simulink model "P1s1"  (R2015b)
settings: Solver=VariableStepAuto  StartTime=0.0  StopTime=10.0  RelTol=1e-3
settings Model: Creator=xmax1946  LastModifiedBy=xmax1946

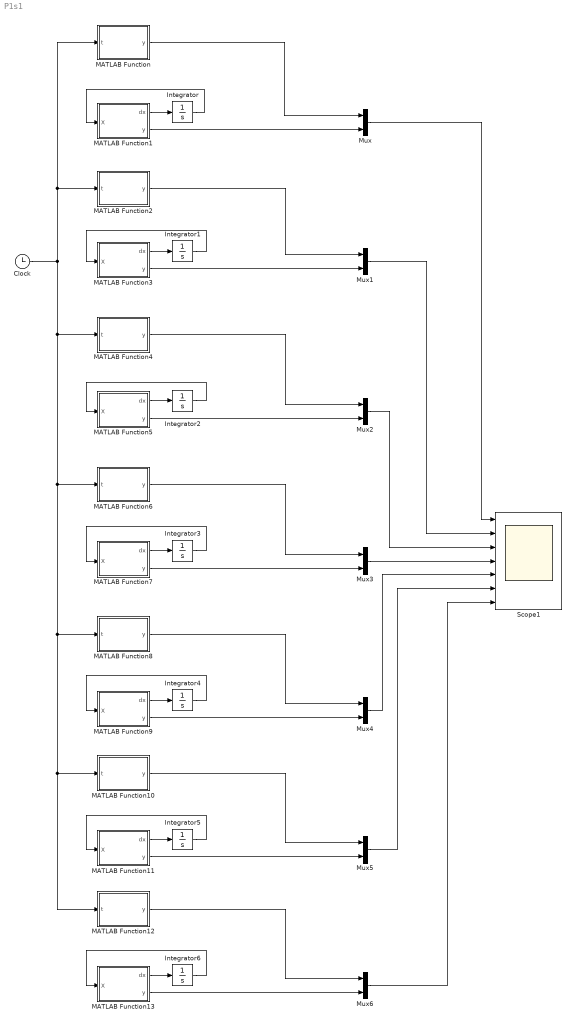
== system P1s1 ==
  Clock : Clock
  Integrator{,1..4} (5 alike) : Integrator  InitialCondition=[1;1]
  Integrator5 : Integrator  InitialCondition=[1;1;1]
  Integrator6 : Integrator  InitialCondition=[1;1;1]
  MATLAB Function : MATLAB Function  TreatAsAtomicUnit=on
  MATLAB Function1 : MATLAB Function  TreatAsAtomicUnit=on
  MATLAB Function10 : MATLAB Function  TreatAsAtomicUnit=on
  MATLAB Function11 : MATLAB Function  TreatAsAtomicUnit=on
  MATLAB Function12 : MATLAB Function  TreatAsAtomicUnit=on
  MATLAB Function13 : MATLAB Function  TreatAsAtomicUnit=on
  MATLAB Function2 : MATLAB Function  TreatAsAtomicUnit=on
  MATLAB Function3 : MATLAB Function  TreatAsAtomicUnit=on
  MATLAB Function4 : MATLAB Function  TreatAsAtomicUnit=on
  MATLAB Function5 : MATLAB Function  TreatAsAtomicUnit=on
  MATLAB Function6 : MATLAB Function  TreatAsAtomicUnit=on
  MATLAB Function7 : MATLAB Function  TreatAsAtomicUnit=on
  MATLAB Function8 : MATLAB Function  TreatAsAtomicUnit=on
  MATLAB Function9 : MATLAB Function  TreatAsAtomicUnit=on
  Mux{,1..6} (7 alike) : Mux  Inputs=2
  Scope1 : Scope  NumInputPorts=7
  wires:
  Integrator/1 -> MATLAB Function1/1(X)
  Clock/1 -> MATLAB Function12/1(t), MATLAB Function10/1(t), MATLAB Function8/1(t), MATLAB Function6/1(t), MATLAB Function4/1(t), MATLAB Function2/1(t), MATLAB Function/1(t)
  MATLAB Function1/1(dx) -> Integrator/1
  MATLAB Function3/1(dx) -> Integrator1/1
  Integrator1/1 -> MATLAB Function3/1(X)
  Mux/1 -> Scope1/1
  MATLAB Function3/2(y) -> Mux1/2
  MATLAB Function2/1(y) -> Mux1/1
  MATLAB Function1/2(y) -> Mux/2
  MATLAB Function/1(y) -> Mux/1
  Mux1/1 -> Scope1/2
  MATLAB Function5/1(dx) -> Integrator2/1
  Integrator2/1 -> MATLAB Function5/1(X)
  MATLAB Function5/2(y) -> Mux2/2
  MATLAB Function4/1(y) -> Mux2/1
  Mux2/1 -> Scope1/3
  MATLAB Function7/1(dx) -> Integrator3/1
  Integrator3/1 -> MATLAB Function7/1(X)
  MATLAB Function7/2(y) -> Mux3/2
  MATLAB Function6/1(y) -> Mux3/1
  Mux3/1 -> Scope1/4
  MATLAB Function9/1(dx) -> Integrator4/1
  Integrator4/1 -> MATLAB Function9/1(X)
  MATLAB Function9/2(y) -> Mux4/2
  MATLAB Function8/1(y) -> Mux4/1
  Mux4/1 -> Scope1/5
  MATLAB Function11/1(dx) -> Integrator5/1
  Integrator5/1 -> MATLAB Function11/1(X)
  MATLAB Function11/2(y) -> Mux5/2
  MATLAB Function10/1(y) -> Mux5/1
  Mux5/1 -> Scope1/6
  MATLAB Function13/1(dx) -> Integrator6/1
  Integrator6/1 -> MATLAB Function13/1(X)
  MATLAB Function13/2(y) -> Mux6/2
  MATLAB Function12/1(y) -> Mux6/1
  Mux6/1 -> Scope1/7

== matlab function P1s1/MATLAB Function1 ==
  data: dx output; X input; y output
function [dx,y] = fcn1(X)

A=[1,-1;0,-1];
B=[1;1];
C=[1,2];
u=1;
dx=A*X+B*u;
y=C*X;

== matlab function P1s1/MATLAB Function ==
  data: t input; y output
function y = f1(t)
y = exp(t)+2;

== matlab function P1s1/MATLAB Function2 ==
  data: t input; y output
function y = f2(t)
y = 11/4 - (25*exp(-4*t))/12 - (2*exp(-t))/3;

== matlab function P1s1/MATLAB Function3 ==
  data: dx output; X input; y output
function [dx,y] = fcn2(X)

A=[0,1;-4,-5];
B=[1;2];
C=[1,-1];
u=1;
dx=A*X+B*u;
y=C*X;

== matlab function P1s1/MATLAB Function4 ==
  data: t input; y output
function y = f3(t)
y = t*exp(-3*t) - (4*exp(-3*t))/3 + 10/3;

== matlab function P1s1/MATLAB Function5 ==
  data: dx output; X input; y output
function [dx,y] = fcn3(X)

A=[-3,1;0,-3];
B=[1;0];
C=[1,1];
u=10;
dx=A*X+B*u;
y=C*X;

== matlab function P1s1/MATLAB Function6 ==
  data: t input; y output
function y = f4(t)
y =5/3 - exp(-4*t) - (2*exp(-3*t))/3;

== matlab function P1s1/MATLAB Function7 ==
  data: dx output; X input; y output
function [dx,y] = fcn4(X)

A=[-4,0;0,-3];
B=[0;1];
C=[-1,1];
u=5;
dx=A*X+B*u;
y=C*X;

== matlab function P1s1/MATLAB Function8 ==
  data: t input; y output
function y = f5(t)
y =33*exp(-t) - 12*exp(-2*t) - 20;

== matlab function P1s1/MATLAB Function9 ==
  data: dx output; X input; y output
function [dx,y] = fcn5(X)

A=[0,1;-2,-3];
B=[1;1];
C=[1,0];
u=-10;
dx=A*X+B*u;
y=C*X;

== matlab function P1s1/MATLAB Function10 ==
  data: t input; y output
function y = f6(t)
y =1 - exp(-2*t);

== matlab function P1s1/MATLAB Function11 ==
  data: dx output; X input; y output
function [dx,y] = fcn6(X)

A=[-1,0,0;0,-2,1;0,0,-2];
B=[1;1;0];
C=[1,0,-1];
u=1;
dx=A*X+B*u;
y=C*X;

== matlab function P1s1/MATLAB Function12 ==
  data: t input; y output
function y = f7(t)
y =(219*exp(-5*t))/125 + (44*t*exp(-5*t))/25 + (2*t^2*exp(-5*t))/5 + 31/125;

== matlab function P1s1/MATLAB Function13 ==
  data: dx output; X input; y output
function [dx,y] = fcn6(X)

A=[-5,1,0;0,-5,1;0,0,-5];
B=[1;0;1];
C=[1,1,0];
u=1;
dx=A*X+B*u;
y=C*X;
